simulink model "simulink_resolution"  (R2019b)
settings: Solver=ode23t  StartTime=0.0  StopTime=5  RelTol=1e-3
values from neighbouring files (symbols this model uses):
  b = 2    [F_mass_spring_damper.m]    (also in mass_spring_damper_parameters.m; ode_solve_mass_spring_damper.m)
  g = 9.81    [F_mass_spring_damper.m]    (also in mass_spring_damper_parameters.m; ode_solve_mass_spring_damper.m)
  k = 100    [F_mass_spring_damper.m]    (also in mass_spring_damper_parameters.m; ode_solve_mass_spring_damper.m)
  m = 1    [F_mass_spring_damper.m]    (also in mass_spring_damper_parameters.m; ode_solve_mass_spring_damper.m)
settings Model: Creator=ivanl  LastModifiedBy=ivanl

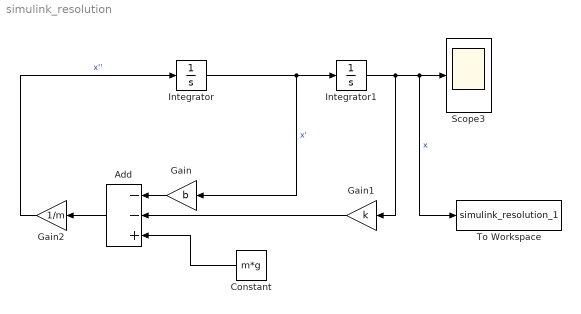
== system simulink_resolution ==
  Add : Sum  Inputs=--+
  Constant : Constant  Value=m*g
  Gain : Gain  Gain=b
  Gain1 : Gain  Gain=k
  Gain2 : Gain  Gain=1/m
  Integrator : Integrator
  Integrator1 : Integrator  InitialCondition=0.1
  Scope3 : Scope
  To Workspace : ToWorkspace  VariableName=simulink_resolution_1  SampleTime=-1
  wires:
  Gain/1 -> Add/1
  Add/1 -> Gain2/1
  Gain1/1 -> Add/2
  Constant/1 -> Add/3
  Integrator1/1 -> To Workspace/1, Scope3/1, Gain1/1  "x"
  Gain2/1 -> Integrator/1  "x''"
  Integrator/1 -> Gain/1, Integrator1/1  "x'"
